simulink model "arduino_serial_gps_standalone"  (R2024b)
settings: Solver=FixedStepAuto  StartTime=0.0  StopTime=10  RelTol=1e-3  EnableMultiTasking=on
libraries: arduinolib x2, realtime_examples_misc x1
settings Model: ExtModeTrigDuration=2  ExtModeArchiveDirName=C:\Users\mmordeka\Desktop\2_6_morning  ExtModeAddSuffixToVar=on  Creator=The MathWorks, Inc.  LastModifiedBy=Nitesh
settings SolverCC: AlgebraicLoopSolver=TrustRegion  AutoInsertRateTranBlk=on
settings DataIOCC: ReturnWorkspaceOutputs=off
settings OptimizationCC: PassReuseOutputArgsThreshold=0  MaxStackSize=64
settings DebuggingCC: ParameterTunabilityLossMsg=error  UnconnectedInputMsg=warning  UnconnectedOutputMsg=warning  UnconnectedLineMsg=warning  ArithmeticOperatorsInVariantConditions=warning
settings HardwareCC: ProdBitPerPointer=32  ProdBitPerSizeT=32  ProdBitPerPtrDiffT=32  ProdLargestAtomicInteger=Long  ProdLargestAtomicFloat=Double  ProdWordSize=32  ProdHWDeviceType=ARM Compatible->ARM Cortex  UseEmbeddedCoderFeatures=off
settings ModelReferenceCC: EnableRefExpFcnMdlSchedulingChecks=on
settings SFSimCC: SimUseLocalCustomCode=off  MATLABDynamicMemAlloc=off  CustomCodeUndefinedFunction=UseInterfaceOnly
settings RTWCC: Description=Embedded Coder  SystemTargetFile=ert.tlc  HardwareBoard=ESP32-WROOM(Arduino Compatible)  TLCOptions="-aInlineSetEventsForThisBaseRateFcn=TLC_FALSE -aSuppressMultiTaskScheduler=TLC_FALSE  -aRateBasedStepFcn=0"  TemplateMakefile=ert_default_tmf  GenerateReport=on  RTWUseLocalCustomCode=off  Toolchain=ESP32  BuildConfiguration=Faster Runs  LaunchReport=on  GPUComputeCapability=3.5
settings CodeAppCC: ForceParamTrailComments=on  OperatorAnnotations=on  StateflowObjectComments=on  MATLABSourceComments=on
settings ERTTargetCC: ERTCustomFileBanners=off  SupportContinuousTime=on  SupportNonInlinedSFcns=on  RemoveResetFunc=off  SupportVariableSizeSignals=on  ModelStepFunctionPrototypeControlCompliant=off  ExtModeTransport=3  ExtModeStaticAlloc=on  ExtModeAutomaticAllocSize=off  ExtModeStaticAllocSize=65536  ExtModeMexFile=ext_xcp  ExtModeIntrfLevel=Level2 - Open  InlinedParameterPlacement=Hierarchical  DynamicArrayContainerType=coder::array

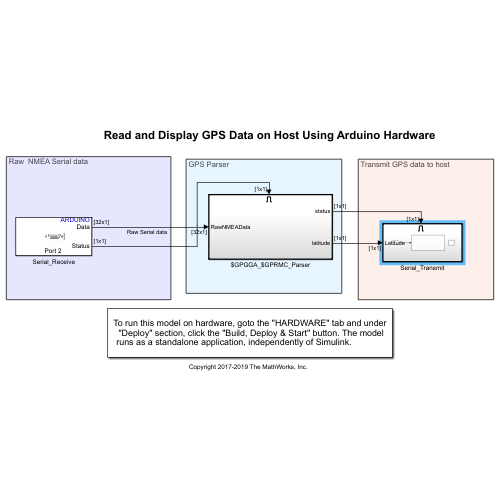
[thumbnail: Simulink's stored preview of the top-level diagram]
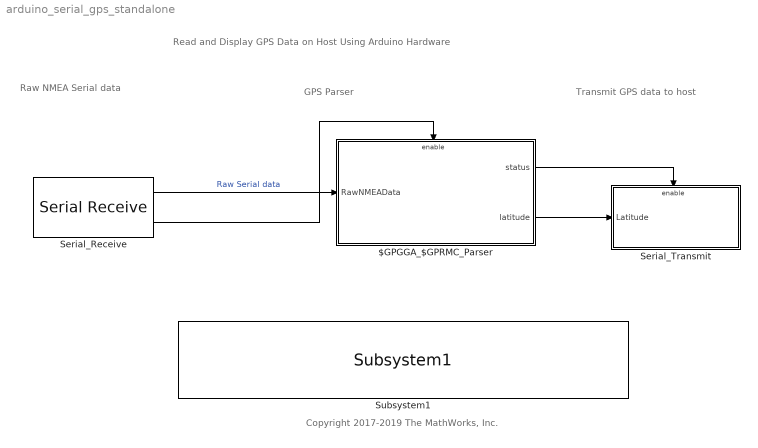
== system arduino_serial_gps_standalone ==
  note: Transmit GPS data to host
  note: GPS Parser
  note: Raw NMEA Serial data
  note: Read and Display GPS Data on Host Using Arduino Hardware
  note: Copyright 2017-2019 The MathWorks, Inc.
  $GPGGA_$GPRMC_Parser : Subsystem  TreatAsAtomicUnit=on
  Serial_Receive : arduinolib/Serial Receive  portNumber=2  DataType=uint8  blockPlatform=arduino  TimeOut=0  MaxDataLength=10  isARMArch=off  DataLengthOption=Length via dialog  Datalength=32  Header=[]  Terminator=[]  SampleTime=0.03  ShowOutStatus=on
      settings: SourceProductName=Common
  Serial_Transmit : Subsystem
  Subsystem1 : realtime_examples_misc/Subsystem1  SystemSampleTime=-1  VariantActivationTime=update diagram  AllowFlexibleInterface=on  Latency=0  AutoFrameSizeCalculation=off
  wires:
  Serial_Receive/1 -> $GPGGA_$GPRMC_Parser/1(RawNMEAData)  "Raw Serial data"
  Serial_Receive/2 -> $GPGGA_$GPRMC_Parser/Enable
  $GPGGA_$GPRMC_Parser/1(status) -> Serial_Transmit/Enable
  $GPGGA_$GPRMC_Parser/2(latitude) -> Serial_Transmit/1(Latitude)

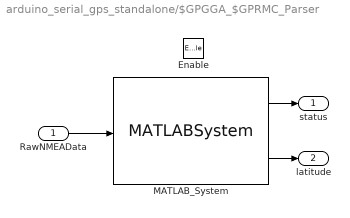
== system arduino_serial_gps_standalone/$GPGGA_$GPRMC_Parser ==
  RawNMEAData : Inport
  Enable : EnablePort  StatesWhenEnabling=reset
  MATLAB_System : MATLABSystem  System=GPSParser  TimeOpt=off  LatOpt=on  LonOpt=off  NoSatOpt=off  HdopOpt=off  AltOpt=off  MslOpt=off  SpeedOpt=off  DateOpt=off  TckAngOpt=off
      mask Type: GPSParser
      mask Display:
      | disp('GPSParser');
      | port_label('input',1,'inData');
      | port_label('output',1,'Status');
      | port_label('output',2,'Latitude');
  status : Outport  OutputWhenDisabled=reset  InitialOutput=0  VectorParamsAs1DForOutWhenUnconnected=off
  latitude : Outport  Port=2  OutputWhenDisabled=reset  InitialOutput=0  VectorParamsAs1DForOutWhenUnconnected=off
  wires:
  MATLAB_System/1 -> status/1
  RawNMEAData/1 -> MATLAB_System/1
  MATLAB_System/2 -> latitude/1

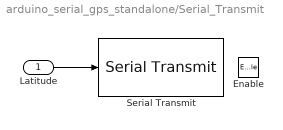
== system arduino_serial_gps_standalone/Serial_Transmit ==
  Latitude : Inport
  Enable : EnablePort
  Serial Transmit : arduinolib/Serial Transmit  portNumber=1  sendmode=println  label=GPS_latitude  sendformat=Decimal  floatprecision=5  header=[]  terminator=[]  blockPlatform=arduino
      settings: SourceProductName=Common
  wires:
  Latitude/1 -> Serial Transmit/1
